simulink model "task_3"  (R2024a)
settings: Solver=VariableStepAuto  StartTime=0.0  StopTime=25  MaxStep=0.001  RelTol=1e-3
undefined symbols (not defined in the file): k
settings Model: Creator=kit  LastModifiedBy=kit

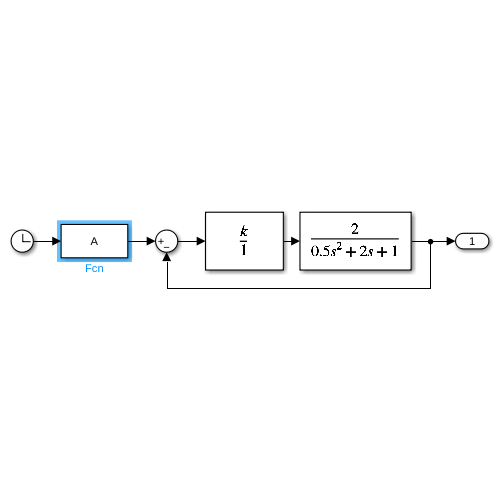
[thumbnail: Simulink's stored preview of the top-level diagram]
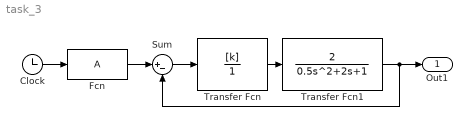
== system task_3 ==
  Clock : Clock
  Fcn : Fcn  Expr=A
  Sum : Sum  Inputs=|+-
  Transfer Fcn : TransferFcn  Numerator=[k]  Denominator=[1]
  Transfer Fcn1 : TransferFcn  Numerator=[2]  Denominator=[0.5 2 1]
  Out1 : Outport
  wires:
  Clock/1 -> Fcn/1
  Fcn/1 -> Sum/1
  Sum/1 -> Transfer Fcn/1
  Transfer Fcn/1 -> Transfer Fcn1/1
  Transfer Fcn1/1 -> Sum/2, Out1/1
